simulink model "vehicle_dynamic_dis_3states"  (R2022b)
settings: Solver=VariableStepAuto  StartTime=0.0  StopTime=9.5  RelTol=1e-3
values from neighbouring files (symbols this model uses):
  A_dis = V_DIS.A    [vehicle_lateral_control_LMIs_3states_auto.m]
  accel = 0.006    [vehicle_lateral_control_LMIs_3states_auto.m]
  B_dis = V_DIS.B    [vehicle_lateral_control_LMIs_3states_auto.m]
  C_dis = V_DIS.C    [vehicle_lateral_control_LMIs_3states_auto.m]
  Cf = 57117    [vehicle_lateral_control_LMIs_3states_auto.m]
  Cr = 81396    [vehicle_lateral_control_LMIs_3states_auto.m]
  D_dis = V_DIS.D    [vehicle_lateral_control_LMIs_3states_auto.m]
  Iz = 1975    [vehicle_lateral_control_LMIs_3states_auto.m]
  K_gain = K_lmi    [vehicle_lateral_control_LMIs_3states_auto.m]
  Ka = value(Ya)*inv(value(P))    [vehicle_lateral_control_LMIs_3states_auto.m]
  Kb = value(Yb)*inv(value(P))    [vehicle_lateral_control_LMIs_3states_auto.m]
  Kc = value(Yc)*inv(value(P))    [vehicle_lateral_control_LMIs_3states_auto.m]
  lf = 1.15    [vehicle_lateral_control_LMIs_3states_auto.m]
  lr = 1.38    [vehicle_lateral_control_LMIs_3states_auto.m]
  m = 1621    [vehicle_lateral_control_LMIs_3states_auto.m]
  Ts = 0.01    [vehicle_lateral_control_LMIs_3states_auto.m]
  vx_track = 15    [vehicle_lateral_control_LMIs_3states_auto.m]
  wp = wpt(L,vx_track)    [vehicle_lateral_control_LMIs_3states_auto.m]
libraries: cstblocks x2
settings Model: Creator=phatdo  LastModifiedBy=phatdo
settings DataIOCC: ReturnWorkspaceOutputs=off

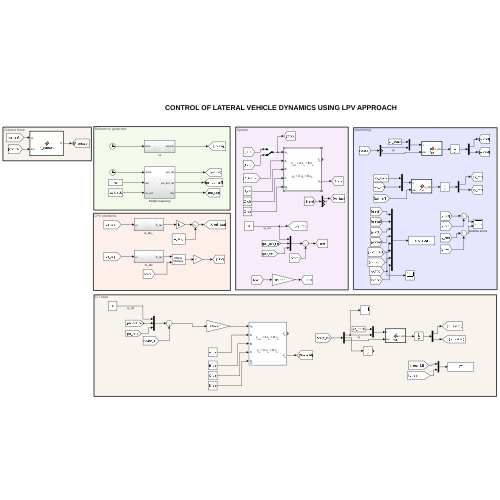
[thumbnail: Simulink's stored preview of the top-level diagram]
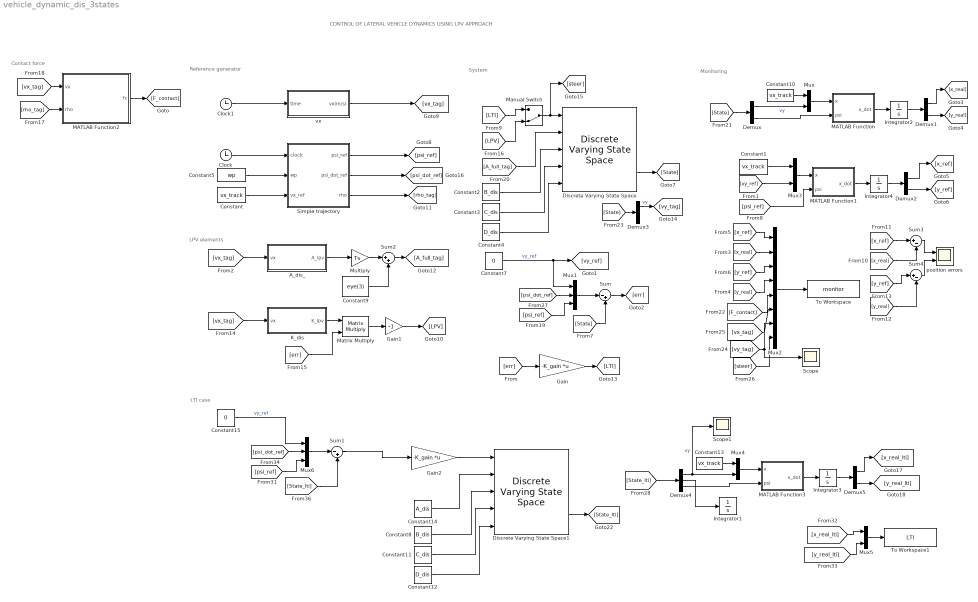
== system vehicle_dynamic_dis_3states ==
  note: LTI case
  note: CONTROL OF LATERAL VEHICLE DYNAMICS USING LPV APPROACH
  note: System
  note: LPV elements
  note: Reference generator
  note: Contact force
  note: Monitoring
  A_dis_ : Subsystem
  Clock : Clock
  Clock1 : Clock
  Constant{,1,10,13} (4 alike) : Constant  Value=vx_track
  Constant11 : Constant  Value=C_dis
  Constant12 : Constant  Value=D_dis
  Constant14 : Constant  Value=A_dis
  Constant15 : Constant  Value=0
  Constant2 : Constant  Value=B_dis
  Constant3 : Constant  Value=C_dis
  Constant4 : Constant  Value=D_dis
  Constant5 : Constant  Value=wp
  Constant7 : Constant  Value=0
  Constant8 : Constant  Value=B_dis
  Constant9 : Constant  Value=eye(3)
  Demux : Demux  Outputs=3
  Demux1 : Demux  Outputs=2
  Demux2 : Demux  Outputs=2
  Demux3 : Demux  Outputs=3
  Demux4 : Demux  Outputs=3
  Demux5 : Demux  Outputs=2
  Discrete Varying State Space : cstblocks/Linear Parameter Varying/Discrete Varying State Space  x0=0  Ts=Ts  OutputX=on  OutputDX=off
  Discrete Varying State Space1 : cstblocks/Linear Parameter Varying/Discrete Varying State Space  x0=0  Ts=Ts  OutputX=on  OutputDX=off
  Gain : Gain  Gain=-K_gain  Multiplication=Matrix(K*u) (u vector)
  Gain1 : Gain  Gain=-1
  Gain2 : Gain  Gain=-K_gain  Multiplication=Matrix(K*u) (u vector)
  Integrator{1..4} (4 alike) : Integrator
  K_dis : Subsystem
  MATLAB Function : MATLAB Function  TreatAsAtomicUnit=on
  MATLAB Function1 : MATLAB Function  TreatAsAtomicUnit=on
  MATLAB Function2 : MATLAB Function  TreatAsAtomicUnit=on
  MATLAB Function3 : MATLAB Function  TreatAsAtomicUnit=on
  Manual Switch : ManualSwitch  CurrentSetting=0
  Matrix Multiply : Product  Multiplication=Matrix(*)
  Multiply : Gain  Gain=Ts
  Mux{,3..5} (4 alike) : Mux  Inputs=2
  Mux1 : Mux  Inputs=3
  Mux2 : Mux  Inputs=8
  Mux6 : Mux  Inputs=3
  Scope : Scope
  Scope1 : Scope
  Simple trajectory : Subsystem
  Sum : Sum  Inputs=|-+
  Sum1 : Sum  Inputs=|-+
  Sum2 : Sum  Inputs=|++
  Sum3 : Sum  Inputs=|+-
  Sum4 : Sum  Inputs=|+-
  To Workspace : ToWorkspace  VariableName=monitor  SaveFormat=Timeseries  SampleTime=-1
  To Workspace1 : ToWorkspace  VariableName=LTI  SaveFormat=Timeseries  SampleTime=-1
  position errors : Scope  NumInputPorts=2
  vx : Subsystem
  wires:
  Demux/1 -> Mux/2  "vy"
  Mux/1 -> MATLAB Function/1(x)
  MATLAB Function/1(x_dot) -> Integrator2/1
  Integrator2/1 -> Demux1/1
  Sum/1 -> [err]
  Mux1/1 -> Sum/1
  Constant7/1 -> [vy_ref], Mux1/1  "vy_ref"
  [vy_ref] -> Mux3/2
  Mux3/1 -> MATLAB Function1/1(x)
  MATLAB Function1/1(x_dot) -> Integrator4/1
  Integrator4/1 -> Demux2/1
  Constant1/1 -> Mux3/1
  [psi_ref] -> MATLAB Function1/2(psi)
  Demux1/1 -> [x_real]
  Demux1/2 -> [y_real]
  Demux2/1 -> [x_ref]
  Demux2/2 -> [y_ref]
  [x_ref] -> Mux2/1
  [x_real] -> Mux2/2
  [y_ref] -> Mux2/3
  [y_real] -> Mux2/4
  Mux2/1 -> To Workspace/1
  Constant2/1 -> Discrete Varying State Space/3
  Constant3/1 -> Discrete Varying State Space/4
  Constant4/1 -> Discrete Varying State Space/5
  Discrete Varying State Space/2 -> [State]
  [State] -> Sum/2
  Constant5/1 -> Simple trajectory/2(wp)
  Clock/1 -> Simple trajectory/1(clock)
  Constant/1 -> Simple trajectory/3(vx_ref)
  [vx_tag] -> A_dis_/1(vx)
  A_dis_/1(A_lpv) -> Multiply/1
  Multiply/1 -> Sum2/1
  Constant9/1 -> Sum2/2
  Simple trajectory/1(psi_ref) -> [psi_ref]
  Sum3/1 -> position errors/1
  Sum4/1 -> position errors/2
  [x_ref] -> Sum3/1
  [x_real] -> Sum3/2
  [y_ref] -> Sum4/1
  [y_real] -> Sum4/2
  K_dis/1(K_lpv) -> Matrix Multiply/1
  [vx_tag] -> K_dis/1(vx)
  [err] -> Matrix Multiply/2
  Matrix Multiply/1 -> Gain1/1
  Gain1/1 -> [LPV]
  Simple trajectory/3(rho) -> [rho_tag]
  [rho_tag] -> MATLAB Function2/2(rho)
  MATLAB Function2/1(fc) -> [F_contact]
  [vx_tag] -> MATLAB Function2/1(vx)
  Sum2/1 -> [A_full_tag]
  [A_full_tag] -> Discrete Varying State Space/2
  [err] -> Gain/1
  Gain/1 -> [LTI]
  [State] -> Demux/1
  Constant10/1 -> Mux/1
  [F_contact] -> Mux2/5
  [State] -> Demux3/1
  Demux3/1 -> [vy_tag]  "vy"
  [vy_tag] -> Mux2/7, Scope/1
  [vx_tag] -> Mux2/6
  Manual Switch/1 -> [steer], Discrete Varying State Space/1
  [LTI] -> Manual Switch/1
  [LPV] -> Manual Switch/2
  [steer] -> Mux2/8
  Simple trajectory/2(psi_dot_ref) -> [psi_dot_ref]
  Demux/3 -> MATLAB Function/2(psi)
  [psi_ref] -> Mux1/3
  [psi_dot_ref] -> Mux1/2
  Clock1/1 -> vx/1(time)
  vx/1(vx(m/s)) -> [vx_tag]
  Gain2/1 -> Discrete Varying State Space1/1
  Constant14/1 -> Discrete Varying State Space1/2
  Discrete Varying State Space1/2 -> [State_lti]
  Constant12/1 -> Discrete Varying State Space1/5
  Constant11/1 -> Discrete Varying State Space1/4
  Constant8/1 -> Discrete Varying State Space1/3
  Demux4/1 -> Scope1/1, Mux4/2  "vy"
  Mux4/1 -> MATLAB Function3/1(x)
  Demux4/2 -> Integrator1/1
  MATLAB Function3/1(x_dot) -> Integrator3/1
  Integrator3/1 -> Demux5/1
  Demux5/2 -> [y_real_lti]
  Demux5/1 -> [x_real_lti]
  Constant13/1 -> Mux4/1
  [State_lti] -> Demux4/1
  Demux4/3 -> MATLAB Function3/2(psi)
  [x_real_lti] -> Mux5/1
  [y_real_lti] -> Mux5/2
  Mux5/1 -> To Workspace1/1
  Mux6/1 -> Sum1/1
  Constant15/1 -> Mux6/1  "vy_ref"
  Sum1/1 -> Gain2/1
  [psi_ref] -> Mux6/3
  [State_lti] -> Sum1/2
  [psi_dot_ref] -> Mux6/2

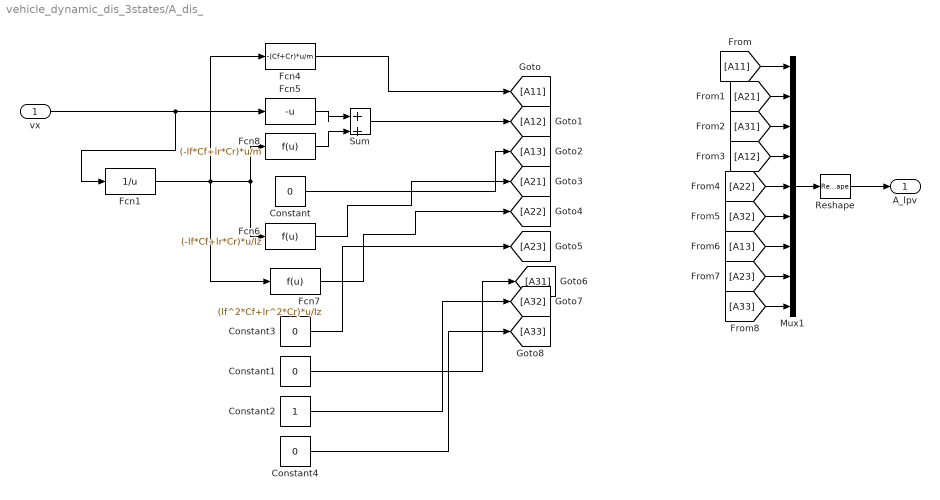
== system vehicle_dynamic_dis_3states/A_dis_ ==
  vx : Inport
  Constant{,1,3..4} (4 alike) : Constant  Value=0
  Constant2 : Constant
  Fcn1 : Fcn  Expr=1/u
  Fcn4 : Fcn  Expr=-(Cf+Cr)*u/m
  Fcn5 : Fcn  Expr=-u
  Fcn6 : Fcn  Expr=(-lf*Cf+lr*Cr)*u/Iz
  Fcn7 : Fcn  Expr=(lf^2*Cf+lr^2*Cr)*u/Iz
  Fcn8 : Fcn  Expr=(-lf*Cf+lr*Cr)*u/m
  Mux1 : Mux  Inputs=9
  Reshape : Reshape  OutputDimensionality=Customize  OutputDimensions=[3;3]
  Sum : Sum  Inputs=|++
  A_lpv : Outport
  wires:
  Reshape/1 -> A_lpv/1
  Fcn4/1 -> [A11]
  Fcn1/1 -> Fcn6/1, Fcn8/1, Fcn7/1, Fcn4/1
  Fcn5/1 -> Sum/1
  Fcn8/1 -> Sum/2
  Sum/1 -> [A12]
  vx/1 -> Fcn1/1, Fcn5/1
  Constant/1 -> [A13]
  Fcn6/1 -> [A21]
  Fcn7/1 -> [A22]
  Constant3/1 -> [A23]
  Constant1/1 -> [A31]
  Constant2/1 -> [A32]
  Constant4/1 -> [A33]
  Mux1/1 -> Reshape/1
  [A11] -> Mux1/1
  [A21] -> Mux1/2
  [A31] -> Mux1/3
  [A12] -> Mux1/4
  [A22] -> Mux1/5
  [A32] -> Mux1/6
  [A13] -> Mux1/7
  [A23] -> Mux1/8
  [A33] -> Mux1/9

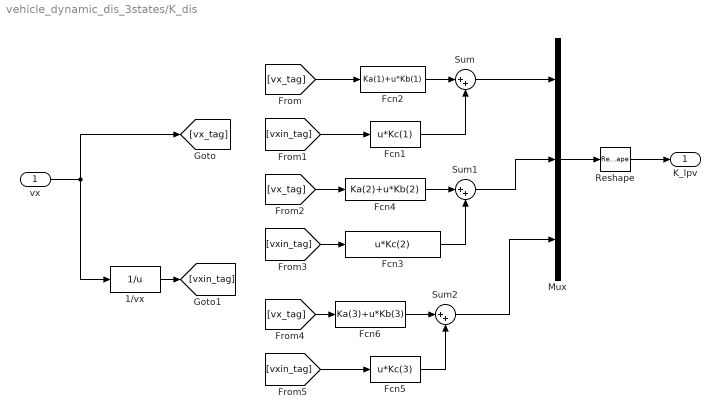
== system vehicle_dynamic_dis_3states/K_dis ==
  vx : Inport
  1/vx : Fcn  Expr=1/u
  Fcn1 : Fcn  Expr=u*Kc(1)
  Fcn2 : Fcn  Expr=Ka(1)+u*Kb(1)
  Fcn3 : Fcn  Expr=u*Kc(2)
  Fcn4 : Fcn  Expr=Ka(2)+u*Kb(2)
  Fcn5 : Fcn  Expr=u*Kc(3)
  Fcn6 : Fcn  Expr=Ka(3)+u*Kb(3)
  Mux : Mux  Inputs=3
  Reshape : Reshape  OutputDimensionality=Customize  OutputDimensions=[1,3]
  Sum : Sum  Inputs=|++
  Sum1 : Sum  Inputs=|++
  Sum2 : Sum  Inputs=|++
  K_lpv : Outport
  wires:
  Mux/1 -> Reshape/1
  Reshape/1 -> K_lpv/1
  vx/1 -> [vx_tag], 1/vx/1
  Fcn2/1 -> Sum/1
  Sum/1 -> Mux/1
  [vx_tag] -> Fcn2/1
  1/vx/1 -> [vxin_tag]
  [vxin_tag] -> Fcn1/1
  Fcn1/1 -> Sum/2
  [vx_tag] -> Fcn4/1
  Fcn3/1 -> Sum1/2
  Sum1/1 -> Mux/2
  Fcn4/1 -> Sum1/1
  [vxin_tag] -> Fcn3/1
  Fcn5/1 -> Sum2/2
  [vx_tag] -> Fcn6/1
  [vxin_tag] -> Fcn5/1
  Fcn6/1 -> Sum2/1
  Sum2/1 -> Mux/3

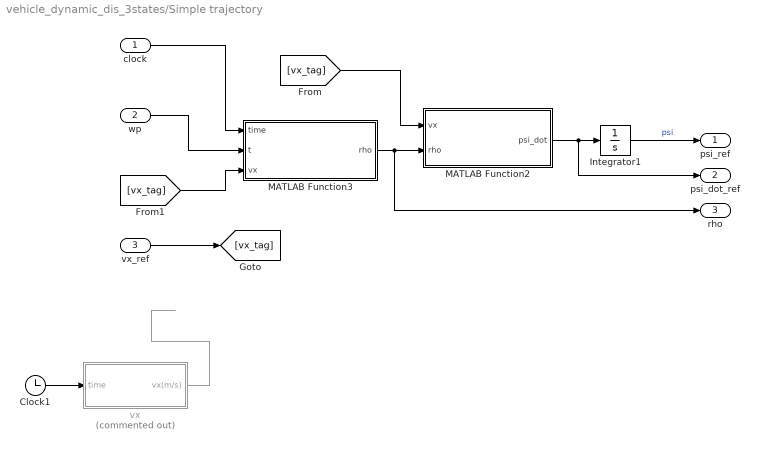
== system vehicle_dynamic_dis_3states/Simple trajectory ==
  clock : Inport
  wp : Inport  Port=2
  vx_ref : Inport  Port=3
  Clock1 : Clock
  Integrator1 : Integrator
  MATLAB Function2 : MATLAB Function  TreatAsAtomicUnit=on
  MATLAB Function3 : MATLAB Function  TreatAsAtomicUnit=on
  vx : Subsystem  Commented=on
  psi_ref : Outport
  psi_dot_ref : Outport  Port=2
  rho : Outport  Port=3
  wires:
  MATLAB Function2/1(psi_dot) -> Integrator1/1, psi_dot_ref/1
  MATLAB Function3/1(rho) -> rho/1, MATLAB Function2/2(rho)
  clock/1 -> MATLAB Function3/1(time)
  wp/1 -> MATLAB Function3/2(t)
  Integrator1/1 -> psi_ref/1  "psi"
  vx_ref/1 -> [vx_tag]
  [vx_tag] -> MATLAB Function2/1(vx)
  [vx_tag] -> MATLAB Function3/3(vx)
  Clock1/1 -> vx/1(time)
  vx/1(vx(m/s)) -> ?

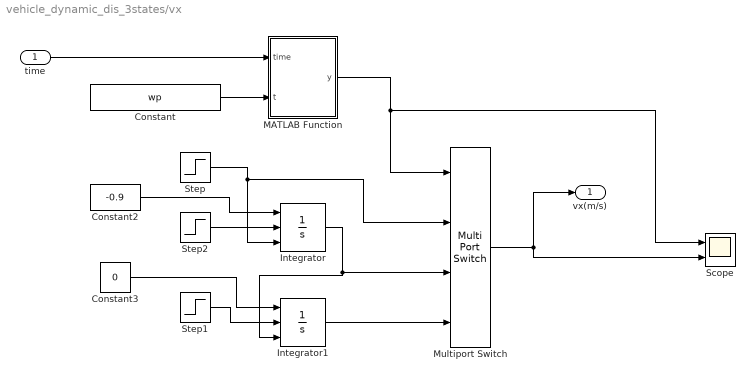
== system vehicle_dynamic_dis_3states/vx ==
  time : Inport
  Constant : Constant  Value=wp
  Constant2 : Constant  Value=-0.9
  Constant3 : Constant  Value=0
  Integrator : Integrator  ExternalReset=rising  InitialConditionSource=external
  Integrator1 : Integrator  ExternalReset=rising  InitialConditionSource=external
  MATLAB Function : MATLAB Function  TreatAsAtomicUnit=on
  Multiport Switch : MultiPortSwitch  SaturateOnIntegerOverflow=off  InputSameDT=off
  Scope : Scope  NumInputPorts=2
  Step : Step  Time=0  Before=14  After=14  SampleTime=0
  Step1 : Step  Time=wp(3)  SampleTime=0
  Step2 : Step  Time=wp(2)  SampleTime=0
  vx(m/s) : Outport
  wires:
  Step/1 -> Integrator/3, Multiport Switch/2
  Constant/1 -> MATLAB Function/2(t)
  Constant2/1 -> Integrator/1
  Multiport Switch/1 -> vx(m/s)/1, Scope/2
  Integrator/1 -> Integrator1/3, Multiport Switch/3
  Step2/1 -> Integrator/2
  Constant3/1 -> Integrator1/1
  Integrator1/1 -> Multiport Switch/4
  Step1/1 -> Integrator1/2
  time/1 -> MATLAB Function/1(time)
  MATLAB Function/1(y) -> Scope/1, Multiport Switch/1

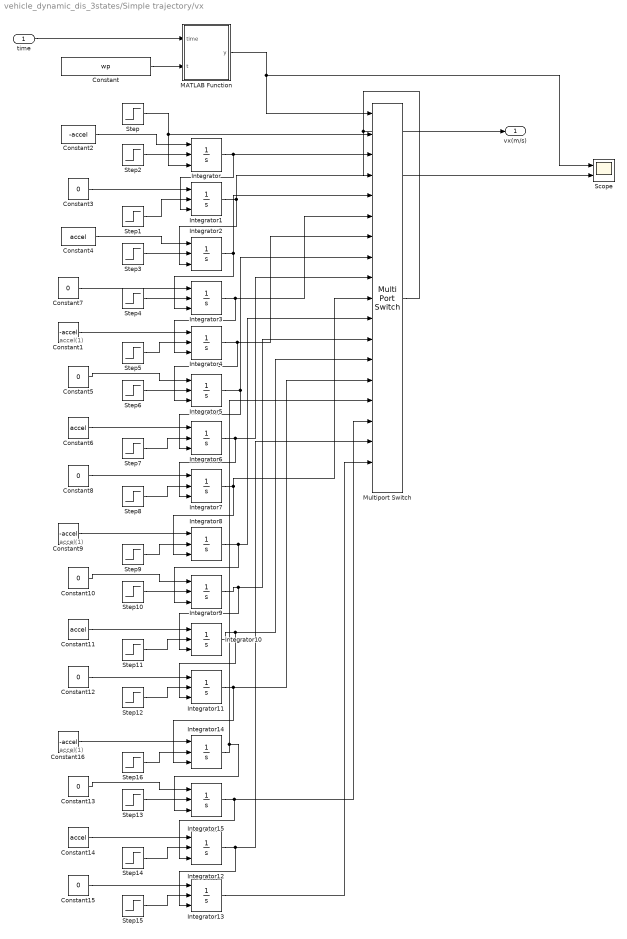
== system vehicle_dynamic_dis_3states/Simple trajectory/vx ==
  note: accel(1)
  note: accel(1)
  note: accel(1)
  time : Inport
  Constant : Constant  Value=wp
  Constant{1..2,9,16} (4 alike) : Constant  Value=-accel
  Constant{3,5,7..8,10,12..13,15} (8 alike) : Constant  Value=0
  Constant{4,6,11,14} (4 alike) : Constant  Value=accel
  Integrator{,1..15} (16 alike) : Integrator  ExternalReset=rising  InitialConditionSource=external
  MATLAB Function : MATLAB Function  TreatAsAtomicUnit=on
  Multiport Switch : MultiPortSwitch  Inputs=18  SaturateOnIntegerOverflow=off  InputSameDT=off
  Scope : Scope  NumInputPorts=2
  Step : Step  Time=0  After=0  SampleTime=0
  Step1 : Step  Time=wp(3)  SampleTime=0
  Step10 : Step  Time=wp(11)  SampleTime=0
  Step11 : Step  Time=wp(12)  SampleTime=0
  Step12 : Step  Time=wp(13)  SampleTime=0
  Step13 : Step  Time=wp(15)  SampleTime=0
  Step14 : Step  Time=wp(16)  SampleTime=0
  Step15 : Step  Time=wp(17)  SampleTime=0
  Step16 : Step  Time=wp(14)  SampleTime=0
  Step2 : Step  Time=wp(2)  SampleTime=0
  Step3 : Step  Time=wp(4)  SampleTime=0
  Step4 : Step  Time=wp(5)  SampleTime=0
  Step5 : Step  Time=wp(6)  SampleTime=0
  Step6 : Step  Time=wp(7)  SampleTime=0
  Step7 : Step  Time=wp(8)  SampleTime=0
  Step8 : Step  Time=wp(9)  SampleTime=0
  Step9 : Step  Time=wp(10)  SampleTime=0
  vx(m/s) : Outport
  wires:
  Step/1 -> Integrator/3, Multiport Switch/2
  Constant/1 -> MATLAB Function/2(t)
  Constant2/1 -> Integrator/1
  Multiport Switch/1 -> Scope/2, vx(m/s)/1
  Integrator/1 -> Integrator1/3, Multiport Switch/3
  Step2/1 -> Integrator/2
  Constant3/1 -> Integrator1/1
  Integrator1/1 -> Integrator2/3, Multiport Switch/4
  Step1/1 -> Integrator1/2
  time/1 -> MATLAB Function/1(time)
  Step3/1 -> Integrator2/2
  Constant4/1 -> Integrator2/1
  Integrator2/1 -> Integrator3/3, Multiport Switch/5
  Integrator3/1 -> Integrator4/3, Multiport Switch/6
  Step4/1 -> Integrator3/2
  Constant7/1 -> Integrator3/1
  MATLAB Function/1(y) -> Scope/1, Multiport Switch/1
  Integrator4/1 -> Integrator5/3, Multiport Switch/7
  Step5/1 -> Integrator4/2
  Step6/1 -> Integrator5/2
  Constant1/1 -> Integrator4/1
  Constant5/1 -> Integrator5/1
  Integrator5/1 -> Integrator6/3, Multiport Switch/8
  Step7/1 -> Integrator6/2
  Constant6/1 -> Integrator6/1
  Constant8/1 -> Integrator7/1
  Step8/1 -> Integrator7/2
  Integrator6/1 -> Integrator7/3, Multiport Switch/9
  Integrator7/1 -> Integrator8/3, Multiport Switch/10
  Constant12/1 -> Integrator11/1
  Constant9/1 -> Integrator8/1
  Constant11/1 -> Integrator10/1
  Step12/1 -> Integrator11/2
  Step11/1 -> Integrator10/2
  Integrator10/1 -> Integrator11/3, Multiport Switch/13
  Step9/1 -> Integrator8/2
  Integrator9/1 -> Integrator10/3, Multiport Switch/12
  Step10/1 -> Integrator9/2
  Constant10/1 -> Integrator9/1
  Integrator8/1 -> Integrator9/3, Multiport Switch/11
  Integrator14/1 -> Integrator15/3, Multiport Switch/15
  Integrator11/1 -> Integrator14/3, Multiport Switch/14
  Step16/1 -> Integrator14/2
  Step15/1 -> Integrator13/2
  Integrator12/1 -> Integrator13/3, Multiport Switch/17
  Constant13/1 -> Integrator15/1
  Step14/1 -> Integrator12/2
  Integrator15/1 -> Multiport Switch/16, Integrator12/3
  Constant15/1 -> Integrator13/1
  Step13/1 -> Integrator15/2
  Constant14/1 -> Integrator12/1
  Constant16/1 -> Integrator14/1
  Integrator13/1 -> Multiport Switch/18

== matlab function vehicle_dynamic_dis_3states/MATLAB Function ==
  data: x input; x_dot output; psi input
function x_dot = fcn(x, psi)

% x = [vx, vy]

x_dot = zeros(2,1);

vx = x(1);
vy = x(2);

x_dot(1) = vx*cos(psi) - vy*sin(psi);
x_dot(2) = vx*sin(psi) + vy*cos(psi);

end

== matlab function vehicle_dynamic_dis_3states/Simple trajectory/MATLAB Function2 ==
  data: vx input; psi_dot output; rho input
function psi_dot = yawrate(vx, rho)
    psi_dot = rho*vx; % Yaw rate
end

== matlab function vehicle_dynamic_dis_3states/MATLAB Function1 ==
  data: x input; x_dot output; psi input
function x_dot = fcn(x, psi)

% x = [vx, vy]

x_dot = zeros(2,1);

vx = x(1);
vy = x(2);

x_dot(1) = vx*cos(psi) - vy*sin(psi);
x_dot(2) = vx*sin(psi) + vy*cos(psi);

end

== matlab function vehicle_dynamic_dis_3states/Simple trajectory/MATLAB Function3 ==
  data: time input; t input; rho output; vx input
function rho = curvature_generator(time,t,vx)

L1 = 40;
L2 = 50;
L3 = 60;

rho = 0;
clothoide_const = 2500;
R = 50;
t1 = 0;
t2 = L1/vx;
t3 = L2/vx;
t4 = L3/vx;

if time >= t(1) && time < t(2)
    rho = 0;% go straight
elseif time >= t(2) && time < t(3)
    rho = -vx*(time - t(2))/clothoide_const; % clothoide cornering
else
    rho = -1/R; % circle cornering
end

end

== matlab function vehicle_dynamic_dis_3states/MATLAB Function2 ==
  data: vx input; fc output; rho input
function fc = F_contact(vx,rho)

m = 1621;

fc = m*vx^2*rho;
end

== matlab function vehicle_dynamic_dis_3states/vx/MATLAB Function ==
  data: time input; t input; y output
function y = fcn(time,t)
t1 = t(1);
t2 = t(2);
t3 = t(3);
t4 = t(4);

if time>t1 && time <= t2
    y = 1;
elseif time>t2 && time <= t3
    y = 2;
else 
    y = 3;
end

== matlab function vehicle_dynamic_dis_3states/Simple trajectory/vx/MATLAB Function ==
  data: time input; t input; y output
function y = fcn(time,t)
t0 = t(1);
t1 = t(2);
t2 = t(3);
t3 = t(4);
t4 = t(5);
t5 = t(6);
t6 = t(7);
t7 = t(8);
t8 = t(9);
t9 = t(10);
t10 = t(11);
t11 = t(12);
t12 = t(13);
t13 = t(14);
t14 = t(15);
t15 = t(16);
t16 = t(17);
t17 = t(18);

if time<=t1
    y = 1;
elseif time>t1 && time <= t2
    y = 2;
elseif time>t2 && time <= t3
    y = 3;
elseif time>t3 && time <= t4
    y = 4;
elseif time>t4 && time <= t5
    y = 5;
elseif time>t5 && time <= t6
    y = 6;
elseif time>t6 && time <= t7
    y = 7;
elseif time>t7 && time <= t8
    y = 8;
elseif time>t8 && time <= t9
    y = 9;
elseif time>t9 && time <= t10
    y = 10;
elseif time>t10 && time <= t11
    y = 11;
elseif time>t11 && time <= t12
    y = 12;
elseif time>t12 && time <= t13
    y = 13;
elseif time>t13 && time <= t14
    y = 14;
elseif time>t14 && time <= t15
    y = 15;
elseif time>t15 && time <= t16
    y = 16;
elseif time>t16 && time <= t17
    y = 17;
else 
    y = 18;
end

== matlab function vehicle_dynamic_dis_3states/MATLAB Function3 ==
  data: x input; x_dot output; psi input
function x_dot = fcn(x, psi)

% x = [vx, vy]

x_dot = zeros(2,1);

vx = x(1);
vy = x(2);

x_dot(1) = vx*cos(psi) - vy*sin(psi);
x_dot(2) = vx*sin(psi) + vy*cos(psi);

end
